simulink model "onelink_simscape"  (R2025a)
settings: Solver=ode15s  StartTime=0.0  StopTime=10  RelTol=1e-4
libraries: fl_lib x179, ee_lib x62, nesl_utility x15
(part 2 of 2)

== system onelink_simscape/inverter5 ==
  Electrical Reference1 : fl_lib/Electrical/Electrical Elements/Electrical Reference
  OP2 : ee_lib/Integrated Circuits/Band-Limited Op-Amp  A=1.8E6  Rin=4e6 Ohm  Rout=70 Ohm  Vmin=-24 V  Vmax=24 V  Vdotmax=2.8E6 V/s  f=8E6 Hz  V0=0 V
  m1 : fl_lib/Electrical/Electrical Elements/Resistor  R=1E3 Ohm  i_specify=off  i_priority=None  i=0 A  i_nominal_specify=off  i_nominal_value=1  i_nominal_unit=A  v_specify=off  v_priority=None  v=0 V  v_nominal_specify=off  v_nominal_value=1  v_nominal_unit=V
  m2 : fl_lib/Electrical/Electrical Elements/Resistor  R=1E3 Ohm  i_specify=off  i_priority=None  i=0 A  i_nominal_specify=off  i_nominal_value=1  i_nominal_unit=A  v_specify=off  v_priority=None  v=0 V  v_nominal_specify=off  v_nominal_value=1  v_nominal_unit=V
  in : PMIOPort  Side=Left
  out : PMIOPort  Port=2  Side=Right
  connections:
  m1/LConn1 -- in/RConn1
  out/RConn1 -- OP2/RConn1 -- m2/LConn1
  OP2/LConn2 -- m1/RConn1 -- m2/RConn1
  OP2/LConn1 -- Electrical Reference1/LConn1

== system onelink_simscape/inverter6 ==
  Electrical Reference1 : fl_lib/Electrical/Electrical Elements/Electrical Reference
  OP2 : ee_lib/Integrated Circuits/Band-Limited Op-Amp  A=1.8E6  Rin=4e6 Ohm  Rout=70 Ohm  Vmin=-24 V  Vmax=24 V  Vdotmax=2.8E6 V/s  f=8E6 Hz  V0=0 V
  m1 : fl_lib/Electrical/Electrical Elements/Resistor  R=1E3 Ohm  i_specify=off  i_priority=None  i=0 A  i_nominal_specify=off  i_nominal_value=1  i_nominal_unit=A  v_specify=off  v_priority=None  v=0 V  v_nominal_specify=off  v_nominal_value=1  v_nominal_unit=V
  m2 : fl_lib/Electrical/Electrical Elements/Resistor  R=1E3 Ohm  i_specify=off  i_priority=None  i=0 A  i_nominal_specify=off  i_nominal_value=1  i_nominal_unit=A  v_specify=off  v_priority=None  v=0 V  v_nominal_specify=off  v_nominal_value=1  v_nominal_unit=V
  in : PMIOPort  Side=Left
  out : PMIOPort  Port=2  Side=Right
  connections:
  m1/LConn1 -- in/RConn1
  out/RConn1 -- OP2/RConn1 -- m2/LConn1
  OP2/LConn2 -- m1/RConn1 -- m2/RConn1
  OP2/LConn1 -- Electrical Reference1/LConn1

== system onelink_simscape/inverter7 ==
  Electrical Reference1 : fl_lib/Electrical/Electrical Elements/Electrical Reference
  OP2 : ee_lib/Integrated Circuits/Band-Limited Op-Amp  A=1.8E6  Rin=4e6 Ohm  Rout=70 Ohm  Vmin=-24 V  Vmax=24 V  Vdotmax=2.8E6 V/s  f=8E6 Hz  V0=0 V
  m1 : fl_lib/Electrical/Electrical Elements/Resistor  R=1E3 Ohm  i_specify=off  i_priority=None  i=0 A  i_nominal_specify=off  i_nominal_value=1  i_nominal_unit=A  v_specify=off  v_priority=None  v=0 V  v_nominal_specify=off  v_nominal_value=1  v_nominal_unit=V
  m2 : fl_lib/Electrical/Electrical Elements/Resistor  R=1E3 Ohm  i_specify=off  i_priority=None  i=0 A  i_nominal_specify=off  i_nominal_value=1  i_nominal_unit=A  v_specify=off  v_priority=None  v=0 V  v_nominal_specify=off  v_nominal_value=1  v_nominal_unit=V
  in : PMIOPort  Side=Left
  out : PMIOPort  Port=2  Side=Right
  connections:
  m1/LConn1 -- in/RConn1
  out/RConn1 -- OP2/RConn1 -- m2/LConn1
  OP2/LConn2 -- m1/RConn1 -- m2/RConn1
  OP2/LConn1 -- Electrical Reference1/LConn1

== system onelink_simscape/inverter8 ==
  Electrical Reference1 : fl_lib/Electrical/Electrical Elements/Electrical Reference
  OP2 : ee_lib/Integrated Circuits/Band-Limited Op-Amp  A=1.8E6  Rin=4e6 Ohm  Rout=70 Ohm  Vmin=-24 V  Vmax=24 V  Vdotmax=2.8E6 V/s  f=8E6 Hz  V0=0 V
  m1 : fl_lib/Electrical/Electrical Elements/Resistor  R=1E3 Ohm  i_specify=off  i_priority=None  i=0 A  i_nominal_specify=off  i_nominal_value=1  i_nominal_unit=A  v_specify=off  v_priority=None  v=0 V  v_nominal_specify=off  v_nominal_value=1  v_nominal_unit=V
  m2 : fl_lib/Electrical/Electrical Elements/Resistor  R=1E3 Ohm  i_specify=off  i_priority=None  i=0 A  i_nominal_specify=off  i_nominal_value=1  i_nominal_unit=A  v_specify=off  v_priority=None  v=0 V  v_nominal_specify=off  v_nominal_value=1  v_nominal_unit=V
  in : PMIOPort  Side=Left
  out : PMIOPort  Port=2  Side=Right
  connections:
  m1/LConn1 -- in/RConn1
  out/RConn1 -- OP2/RConn1 -- m2/LConn1
  OP2/LConn2 -- m1/RConn1 -- m2/RConn1
  OP2/LConn1 -- Electrical Reference1/LConn1

== system onelink_simscape/inverter9 ==
  Electrical Reference1 : fl_lib/Electrical/Electrical Elements/Electrical Reference
  OP2 : ee_lib/Integrated Circuits/Band-Limited Op-Amp  A=1.8E6  Rin=4e6 Ohm  Rout=70 Ohm  Vmin=-24 V  Vmax=24 V  Vdotmax=2.8E6 V/s  f=8E6 Hz  V0=0 V
  m1 : fl_lib/Electrical/Electrical Elements/Resistor  R=1E3 Ohm  i_specify=off  i_priority=None  i=0 A  i_nominal_specify=off  i_nominal_value=1  i_nominal_unit=A  v_specify=off  v_priority=None  v=0 V  v_nominal_specify=off  v_nominal_value=1  v_nominal_unit=V
  m2 : fl_lib/Electrical/Electrical Elements/Resistor  R=1E3 Ohm  i_specify=off  i_priority=None  i=0 A  i_nominal_specify=off  i_nominal_value=1  i_nominal_unit=A  v_specify=off  v_priority=None  v=0 V  v_nominal_specify=off  v_nominal_value=1  v_nominal_unit=V
  in : PMIOPort  Side=Left
  out : PMIOPort  Port=2  Side=Right
  connections:
  m1/LConn1 -- in/RConn1
  out/RConn1 -- OP2/RConn1 -- m2/LConn1
  OP2/LConn2 -- m1/RConn1 -- m2/RConn1
  OP2/LConn1 -- Electrical Reference1/LConn1

== system onelink_simscape/mulitplier1 ==
  note: Multiplication circuit. The output voltage is
      | Vx * Vy / K where Multiplier block
      | parameter K is the scaling factor.
  ERef M1Y1 : fl_lib/Electrical/Electrical Elements/Electrical Reference
  ERef M1Y2 : fl_lib/Electrical/Electrical Elements/Electrical Reference
  ERef M1Z2 : fl_lib/Electrical/Electrical Elements/Electrical Reference
  Multiplier 1 : ee_lib/Integrated Circuits/Multiplier  K=1 V  A=3e+3  Rin=1e+7 Ohm  Vdiff=24 V  Rout=0.1 Ohm  Vmin=-11 V  Vmax=11 V  Vdotmax=20 V/us  f=1 MHz  V0=0 V
      settings: AttributesFormatString=Scaling Factor = %<K>  InternalSimscapePortConfiguration="{\"Bottom\":[],\"Left\":[{\"id\":\"X1\",\"label\":\"X1\",\"type\":\"foundation.electrical.electrical\"},{\"id\":\"X2\",\"label\":\"X2\",\"type\":\"foundation.electrical.electrical\"},{\"id\":\"Y1\",\"label\":\"Y1\",\"type\":\"foundation.electrical.electrical\"},{\"id\":\"Y2\",\"label\":\"Y2\",\"type\":\"foundation.electrical.electrical\"},{\"id\":\"Z1\",\"label\":\"Z1\",\"type\":\"foundation.electrical.electrical\"},{\"id\":\"Z2\",\"label\":\"Z2\",\"type\":\"foundation.electrical.electrical\"}],\"Right\":[{\"id\":\"out\",\"label\":\"\",\"type\":\"foundation.electrical.electrical\"}],\"Top\":[]}"
  in1 : PMIOPort  Side=Left
  in2 : PMIOPort  Port=2  Side=Left
  out : PMIOPort  Port=3  Side=Right
  connections:
  Multiplier 1/RConn1 -- out/RConn1 -- Multiplier 1/LConn5
  ERef M1Z2/LConn1 -- Multiplier 1/LConn6
  ERef M1Y2/LConn1 -- Multiplier 1/LConn4
  Multiplier 1/LConn3 -- in2/RConn1
  Multiplier 1/LConn2 -- ERef M1Y1/LConn1
  Multiplier 1/LConn1 -- in1/RConn1

== system onelink_simscape/mulitplier10 ==
  note: Multiplication circuit. The output voltage is
      | Vx * Vy / K where Multiplier block
      | parameter K is the scaling factor.
  ERef M1Y1 : fl_lib/Electrical/Electrical Elements/Electrical Reference
  ERef M1Y2 : fl_lib/Electrical/Electrical Elements/Electrical Reference
  ERef M1Z2 : fl_lib/Electrical/Electrical Elements/Electrical Reference
  Multiplier 1 : ee_lib/Integrated Circuits/Multiplier  K=1 V  A=3e+3  Rin=1e+7 Ohm  Vdiff=10 V  Rout=0.1 Ohm  Vmin=-11 V  Vmax=11 V  Vdotmax=20 V/us  f=1 MHz  V0=0 V
      settings: AttributesFormatString=Scaling Factor = %<K>  InternalSimscapePortConfiguration="{\"Bottom\":[],\"Left\":[{\"id\":\"X1\",\"label\":\"X1\",\"type\":\"foundation.electrical.electrical\"},{\"id\":\"X2\",\"label\":\"X2\",\"type\":\"foundation.electrical.electrical\"},{\"id\":\"Y1\",\"label\":\"Y1\",\"type\":\"foundation.electrical.electrical\"},{\"id\":\"Y2\",\"label\":\"Y2\",\"type\":\"foundation.electrical.electrical\"},{\"id\":\"Z1\",\"label\":\"Z1\",\"type\":\"foundation.electrical.electrical\"},{\"id\":\"Z2\",\"label\":\"Z2\",\"type\":\"foundation.electrical.electrical\"}],\"Right\":[{\"id\":\"out\",\"label\":\"\",\"type\":\"foundation.electrical.electrical\"}],\"Top\":[]}"
  in1 : PMIOPort  Side=Left
  in2 : PMIOPort  Port=2  Side=Left
  out : PMIOPort  Port=3  Side=Right
  connections:
  Multiplier 1/RConn1 -- out/RConn1 -- Multiplier 1/LConn5
  ERef M1Z2/LConn1 -- Multiplier 1/LConn6
  ERef M1Y2/LConn1 -- Multiplier 1/LConn4
  Multiplier 1/LConn3 -- in2/RConn1
  Multiplier 1/LConn2 -- ERef M1Y1/LConn1
  Multiplier 1/LConn1 -- in1/RConn1

== system onelink_simscape/mulitplier11 ==
  note: Multiplication circuit. The output voltage is
      | Vx * Vy / K where Multiplier block
      | parameter K is the scaling factor.
  ERef M1Y1 : fl_lib/Electrical/Electrical Elements/Electrical Reference
  ERef M1Y2 : fl_lib/Electrical/Electrical Elements/Electrical Reference
  ERef M1Z2 : fl_lib/Electrical/Electrical Elements/Electrical Reference
  Multiplier 1 : ee_lib/Integrated Circuits/Multiplier  K=1 V  A=3e+3  Rin=1e+7 Ohm  Vdiff=10 V  Rout=0.1 Ohm  Vmin=-11 V  Vmax=11 V  Vdotmax=20 V/us  f=1 MHz  V0=0 V
      settings: AttributesFormatString=Scaling Factor = %<K>  InternalSimscapePortConfiguration="{\"Bottom\":[],\"Left\":[{\"id\":\"X1\",\"label\":\"X1\",\"type\":\"foundation.electrical.electrical\"},{\"id\":\"X2\",\"label\":\"X2\",\"type\":\"foundation.electrical.electrical\"},{\"id\":\"Y1\",\"label\":\"Y1\",\"type\":\"foundation.electrical.electrical\"},{\"id\":\"Y2\",\"label\":\"Y2\",\"type\":\"foundation.electrical.electrical\"},{\"id\":\"Z1\",\"label\":\"Z1\",\"type\":\"foundation.electrical.electrical\"},{\"id\":\"Z2\",\"label\":\"Z2\",\"type\":\"foundation.electrical.electrical\"}],\"Right\":[{\"id\":\"out\",\"label\":\"\",\"type\":\"foundation.electrical.electrical\"}],\"Top\":[]}"
  in1 : PMIOPort  Side=Left
  in2 : PMIOPort  Port=2  Side=Left
  out : PMIOPort  Port=3  Side=Right
  connections:
  Multiplier 1/RConn1 -- out/RConn1 -- Multiplier 1/LConn5
  ERef M1Z2/LConn1 -- Multiplier 1/LConn6
  ERef M1Y2/LConn1 -- Multiplier 1/LConn4
  Multiplier 1/LConn3 -- in2/RConn1
  Multiplier 1/LConn2 -- ERef M1Y1/LConn1
  Multiplier 1/LConn1 -- in1/RConn1

== system onelink_simscape/mulitplier2 ==
  note: Multiplication circuit. The output voltage is
      | Vx * Vy / K where Multiplier block
      | parameter K is the scaling factor.
  ERef M1Y1 : fl_lib/Electrical/Electrical Elements/Electrical Reference
  ERef M1Y2 : fl_lib/Electrical/Electrical Elements/Electrical Reference
  ERef M1Z2 : fl_lib/Electrical/Electrical Elements/Electrical Reference
  Multiplier 1 : ee_lib/Integrated Circuits/Multiplier  K=1 V  A=3e+3  Rin=1e+7 Ohm  Vdiff=24 V  Rout=0.1 Ohm  Vmin=-11 V  Vmax=11 V  Vdotmax=20 V/us  f=1 MHz  V0=0 V
      settings: AttributesFormatString=Scaling Factor = %<K>  InternalSimscapePortConfiguration="{\"Bottom\":[],\"Left\":[{\"id\":\"X1\",\"label\":\"X1\",\"type\":\"foundation.electrical.electrical\"},{\"id\":\"X2\",\"label\":\"X2\",\"type\":\"foundation.electrical.electrical\"},{\"id\":\"Y1\",\"label\":\"Y1\",\"type\":\"foundation.electrical.electrical\"},{\"id\":\"Y2\",\"label\":\"Y2\",\"type\":\"foundation.electrical.electrical\"},{\"id\":\"Z1\",\"label\":\"Z1\",\"type\":\"foundation.electrical.electrical\"},{\"id\":\"Z2\",\"label\":\"Z2\",\"type\":\"foundation.electrical.electrical\"}],\"Right\":[{\"id\":\"out\",\"label\":\"\",\"type\":\"foundation.electrical.electrical\"}],\"Top\":[]}"
  in1 : PMIOPort  Side=Left
  in2 : PMIOPort  Port=2  Side=Left
  out : PMIOPort  Port=3  Side=Right
  connections:
  Multiplier 1/RConn1 -- out/RConn1 -- Multiplier 1/LConn5
  ERef M1Z2/LConn1 -- Multiplier 1/LConn6
  ERef M1Y2/LConn1 -- Multiplier 1/LConn4
  Multiplier 1/LConn3 -- in2/RConn1
  Multiplier 1/LConn2 -- ERef M1Y1/LConn1
  Multiplier 1/LConn1 -- in1/RConn1

== system onelink_simscape/mulitplier3 ==
  note: Multiplication circuit. The output voltage is
      | Vx * Vy / K where Multiplier block
      | parameter K is the scaling factor.
  ERef M1Y1 : fl_lib/Electrical/Electrical Elements/Electrical Reference
  ERef M1Y2 : fl_lib/Electrical/Electrical Elements/Electrical Reference
  ERef M1Z2 : fl_lib/Electrical/Electrical Elements/Electrical Reference
  Multiplier 1 : ee_lib/Integrated Circuits/Multiplier  K=1 V  A=3e+3  Rin=1e+7 Ohm  Vdiff=24 V  Rout=0.1 Ohm  Vmin=-18 V  Vmax=18 V  Vdotmax=20 V/us  f=1 MHz  V0=0 V
      settings: AttributesFormatString=Scaling Factor = %<K>  InternalSimscapePortConfiguration="{\"Bottom\":[],\"Left\":[{\"id\":\"X1\",\"label\":\"X1\",\"type\":\"foundation.electrical.electrical\"},{\"id\":\"X2\",\"label\":\"X2\",\"type\":\"foundation.electrical.electrical\"},{\"id\":\"Y1\",\"label\":\"Y1\",\"type\":\"foundation.electrical.electrical\"},{\"id\":\"Y2\",\"label\":\"Y2\",\"type\":\"foundation.electrical.electrical\"},{\"id\":\"Z1\",\"label\":\"Z1\",\"type\":\"foundation.electrical.electrical\"},{\"id\":\"Z2\",\"label\":\"Z2\",\"type\":\"foundation.electrical.electrical\"}],\"Right\":[{\"id\":\"out\",\"label\":\"\",\"type\":\"foundation.electrical.electrical\"}],\"Top\":[]}"
  in1 : PMIOPort  Side=Left
  in2 : PMIOPort  Port=2  Side=Left
  out : PMIOPort  Port=3  Side=Right
  connections:
  Multiplier 1/RConn1 -- out/RConn1 -- Multiplier 1/LConn5
  ERef M1Z2/LConn1 -- Multiplier 1/LConn6
  ERef M1Y2/LConn1 -- Multiplier 1/LConn4
  Multiplier 1/LConn3 -- in2/RConn1
  Multiplier 1/LConn2 -- ERef M1Y1/LConn1
  Multiplier 1/LConn1 -- in1/RConn1

== system onelink_simscape/mulitplier4 ==
  note: Multiplication circuit. The output voltage is
      | Vx * Vy / K where Multiplier block
      | parameter K is the scaling factor.
  ERef M1Y1 : fl_lib/Electrical/Electrical Elements/Electrical Reference
  ERef M1Y2 : fl_lib/Electrical/Electrical Elements/Electrical Reference
  ERef M1Z2 : fl_lib/Electrical/Electrical Elements/Electrical Reference
  Multiplier 1 : ee_lib/Integrated Circuits/Multiplier  K=1 V  A=3e+3  Rin=1e+7 Ohm  Vdiff=24 V  Rout=0.1 Ohm  Vmin=-11 V  Vmax=11 V  Vdotmax=20 V/us  f=1 MHz  V0=0 V
      settings: AttributesFormatString=Scaling Factor = %<K>  InternalSimscapePortConfiguration="{\"Bottom\":[],\"Left\":[{\"id\":\"X1\",\"label\":\"X1\",\"type\":\"foundation.electrical.electrical\"},{\"id\":\"X2\",\"label\":\"X2\",\"type\":\"foundation.electrical.electrical\"},{\"id\":\"Y1\",\"label\":\"Y1\",\"type\":\"foundation.electrical.electrical\"},{\"id\":\"Y2\",\"label\":\"Y2\",\"type\":\"foundation.electrical.electrical\"},{\"id\":\"Z1\",\"label\":\"Z1\",\"type\":\"foundation.electrical.electrical\"},{\"id\":\"Z2\",\"label\":\"Z2\",\"type\":\"foundation.electrical.electrical\"}],\"Right\":[{\"id\":\"out\",\"label\":\"\",\"type\":\"foundation.electrical.electrical\"}],\"Top\":[]}"
  in1 : PMIOPort  Side=Left
  in2 : PMIOPort  Port=2  Side=Left
  out : PMIOPort  Port=3  Side=Right
  connections:
  Multiplier 1/RConn1 -- out/RConn1 -- Multiplier 1/LConn5
  ERef M1Z2/LConn1 -- Multiplier 1/LConn6
  ERef M1Y2/LConn1 -- Multiplier 1/LConn4
  Multiplier 1/LConn3 -- in2/RConn1
  Multiplier 1/LConn2 -- ERef M1Y1/LConn1
  Multiplier 1/LConn1 -- in1/RConn1

== system onelink_simscape/mulitplier5 ==
  note: Multiplication circuit. The output voltage is
      | Vx * Vy / K where Multiplier block
      | parameter K is the scaling factor.
  ERef M1Y1 : fl_lib/Electrical/Electrical Elements/Electrical Reference
  ERef M1Y2 : fl_lib/Electrical/Electrical Elements/Electrical Reference
  ERef M1Z2 : fl_lib/Electrical/Electrical Elements/Electrical Reference
  Multiplier 1 : ee_lib/Integrated Circuits/Multiplier  K=1 V  A=3e+3  Rin=1e+7 Ohm  Vdiff=24 V  Rout=0.1 Ohm  Vmin=-11 V  Vmax=11 V  Vdotmax=20 V/us  f=1 MHz  V0=0 V
      settings: AttributesFormatString=Scaling Factor = %<K>  InternalSimscapePortConfiguration="{\"Bottom\":[],\"Left\":[{\"id\":\"X1\",\"label\":\"X1\",\"type\":\"foundation.electrical.electrical\"},{\"id\":\"X2\",\"label\":\"X2\",\"type\":\"foundation.electrical.electrical\"},{\"id\":\"Y1\",\"label\":\"Y1\",\"type\":\"foundation.electrical.electrical\"},{\"id\":\"Y2\",\"label\":\"Y2\",\"type\":\"foundation.electrical.electrical\"},{\"id\":\"Z1\",\"label\":\"Z1\",\"type\":\"foundation.electrical.electrical\"},{\"id\":\"Z2\",\"label\":\"Z2\",\"type\":\"foundation.electrical.electrical\"}],\"Right\":[{\"id\":\"out\",\"label\":\"\",\"type\":\"foundation.electrical.electrical\"}],\"Top\":[]}"
  in1 : PMIOPort  Side=Left
  in2 : PMIOPort  Port=2  Side=Left
  out : PMIOPort  Port=3  Side=Right
  connections:
  Multiplier 1/RConn1 -- out/RConn1 -- Multiplier 1/LConn5
  ERef M1Z2/LConn1 -- Multiplier 1/LConn6
  ERef M1Y2/LConn1 -- Multiplier 1/LConn4
  Multiplier 1/LConn3 -- in2/RConn1
  Multiplier 1/LConn2 -- ERef M1Y1/LConn1
  Multiplier 1/LConn1 -- in1/RConn1

== system onelink_simscape/mulitplier6 ==
  note: Multiplication circuit. The output voltage is
      | Vx * Vy / K where Multiplier block
      | parameter K is the scaling factor.
  ERef M1Y1 : fl_lib/Electrical/Electrical Elements/Electrical Reference
  ERef M1Y2 : fl_lib/Electrical/Electrical Elements/Electrical Reference
  ERef M1Z2 : fl_lib/Electrical/Electrical Elements/Electrical Reference
  Multiplier 1 : ee_lib/Integrated Circuits/Multiplier  K=1 V  A=3e+3  Rin=1e+7 Ohm  Vdiff=24 V  Rout=0.1 Ohm  Vmin=-11 V  Vmax=11 V  Vdotmax=20 V/us  f=1 MHz  V0=0 V
      settings: AttributesFormatString=Scaling Factor = %<K>  InternalSimscapePortConfiguration="{\"Bottom\":[],\"Left\":[{\"id\":\"X1\",\"label\":\"X1\",\"type\":\"foundation.electrical.electrical\"},{\"id\":\"X2\",\"label\":\"X2\",\"type\":\"foundation.electrical.electrical\"},{\"id\":\"Y1\",\"label\":\"Y1\",\"type\":\"foundation.electrical.electrical\"},{\"id\":\"Y2\",\"label\":\"Y2\",\"type\":\"foundation.electrical.electrical\"},{\"id\":\"Z1\",\"label\":\"Z1\",\"type\":\"foundation.electrical.electrical\"},{\"id\":\"Z2\",\"label\":\"Z2\",\"type\":\"foundation.electrical.electrical\"}],\"Right\":[{\"id\":\"out\",\"label\":\"\",\"type\":\"foundation.electrical.electrical\"}],\"Top\":[]}"
  in1 : PMIOPort  Side=Left
  in2 : PMIOPort  Port=2  Side=Left
  out : PMIOPort  Port=3  Side=Right
  connections:
  Multiplier 1/RConn1 -- out/RConn1 -- Multiplier 1/LConn5
  ERef M1Z2/LConn1 -- Multiplier 1/LConn6
  ERef M1Y2/LConn1 -- Multiplier 1/LConn4
  Multiplier 1/LConn3 -- in2/RConn1
  Multiplier 1/LConn2 -- ERef M1Y1/LConn1
  Multiplier 1/LConn1 -- in1/RConn1

== system onelink_simscape/mulitplier7 ==
  note: Multiplication circuit. The output voltage is
      | Vx * Vy / K where Multiplier block
      | parameter K is the scaling factor.
  ERef M1Y1 : fl_lib/Electrical/Electrical Elements/Electrical Reference
  ERef M1Y2 : fl_lib/Electrical/Electrical Elements/Electrical Reference
  ERef M1Z2 : fl_lib/Electrical/Electrical Elements/Electrical Reference
  Multiplier 1 : ee_lib/Integrated Circuits/Multiplier  K=1 V  A=3e+3  Rin=1e+7 Ohm  Vdiff=24 V  Rout=0.1 Ohm  Vmin=-11 V  Vmax=11 V  Vdotmax=20 V/us  f=1 MHz  V0=0 V
      settings: AttributesFormatString=Scaling Factor = %<K>  InternalSimscapePortConfiguration="{\"Bottom\":[],\"Left\":[{\"id\":\"X1\",\"label\":\"X1\",\"type\":\"foundation.electrical.electrical\"},{\"id\":\"X2\",\"label\":\"X2\",\"type\":\"foundation.electrical.electrical\"},{\"id\":\"Y1\",\"label\":\"Y1\",\"type\":\"foundation.electrical.electrical\"},{\"id\":\"Y2\",\"label\":\"Y2\",\"type\":\"foundation.electrical.electrical\"},{\"id\":\"Z1\",\"label\":\"Z1\",\"type\":\"foundation.electrical.electrical\"},{\"id\":\"Z2\",\"label\":\"Z2\",\"type\":\"foundation.electrical.electrical\"}],\"Right\":[{\"id\":\"out\",\"label\":\"\",\"type\":\"foundation.electrical.electrical\"}],\"Top\":[]}"
  in1 : PMIOPort  Side=Left
  in2 : PMIOPort  Port=2  Side=Left
  out : PMIOPort  Port=3  Side=Right
  connections:
  Multiplier 1/RConn1 -- out/RConn1 -- Multiplier 1/LConn5
  ERef M1Z2/LConn1 -- Multiplier 1/LConn6
  ERef M1Y2/LConn1 -- Multiplier 1/LConn4
  Multiplier 1/LConn3 -- in2/RConn1
  Multiplier 1/LConn2 -- ERef M1Y1/LConn1
  Multiplier 1/LConn1 -- in1/RConn1

== system onelink_simscape/mulitplier8 ==
  note: Multiplication circuit. The output voltage is
      | Vx * Vy / K where Multiplier block
      | parameter K is the scaling factor.
  ERef M1Y1 : fl_lib/Electrical/Electrical Elements/Electrical Reference
  ERef M1Y2 : fl_lib/Electrical/Electrical Elements/Electrical Reference
  ERef M1Z2 : fl_lib/Electrical/Electrical Elements/Electrical Reference
  Multiplier 1 : ee_lib/Integrated Circuits/Multiplier  K=1 V  A=3e+3  Rin=1e+7 Ohm  Vdiff=24 V  Rout=0.1 Ohm  Vmin=-11 V  Vmax=11 V  Vdotmax=20 V/us  f=1 MHz  V0=0 V
      settings: AttributesFormatString=Scaling Factor = %<K>  InternalSimscapePortConfiguration="{\"Bottom\":[],\"Left\":[{\"id\":\"X1\",\"label\":\"X1\",\"type\":\"foundation.electrical.electrical\"},{\"id\":\"X2\",\"label\":\"X2\",\"type\":\"foundation.electrical.electrical\"},{\"id\":\"Y1\",\"label\":\"Y1\",\"type\":\"foundation.electrical.electrical\"},{\"id\":\"Y2\",\"label\":\"Y2\",\"type\":\"foundation.electrical.electrical\"},{\"id\":\"Z1\",\"label\":\"Z1\",\"type\":\"foundation.electrical.electrical\"},{\"id\":\"Z2\",\"label\":\"Z2\",\"type\":\"foundation.electrical.electrical\"}],\"Right\":[{\"id\":\"out\",\"label\":\"\",\"type\":\"foundation.electrical.electrical\"}],\"Top\":[]}"
  in1 : PMIOPort  Side=Left
  in2 : PMIOPort  Port=2  Side=Left
  out : PMIOPort  Port=3  Side=Right
  connections:
  Multiplier 1/RConn1 -- out/RConn1 -- Multiplier 1/LConn5
  ERef M1Z2/LConn1 -- Multiplier 1/LConn6
  ERef M1Y2/LConn1 -- Multiplier 1/LConn4
  Multiplier 1/LConn3 -- in2/RConn1
  Multiplier 1/LConn2 -- ERef M1Y1/LConn1
  Multiplier 1/LConn1 -- in1/RConn1

== system onelink_simscape/mulitplier9 ==
  note: Multiplication circuit. The output voltage is
      | Vx * Vy / K where Multiplier block
      | parameter K is the scaling factor.
  ERef M1Y1 : fl_lib/Electrical/Electrical Elements/Electrical Reference
  ERef M1Y2 : fl_lib/Electrical/Electrical Elements/Electrical Reference
  ERef M1Z2 : fl_lib/Electrical/Electrical Elements/Electrical Reference
  Multiplier 1 : ee_lib/Integrated Circuits/Multiplier  K=1 V  A=3e+3  Rin=1e+7 Ohm  Vdiff=24 V  Rout=0.1 Ohm  Vmin=-11 V  Vmax=11 V  Vdotmax=20 V/us  f=1 MHz  V0=0 V
      settings: AttributesFormatString=Scaling Factor = %<K>  InternalSimscapePortConfiguration="{\"Bottom\":[],\"Left\":[{\"id\":\"X1\",\"label\":\"X1\",\"type\":\"foundation.electrical.electrical\"},{\"id\":\"X2\",\"label\":\"X2\",\"type\":\"foundation.electrical.electrical\"},{\"id\":\"Y1\",\"label\":\"Y1\",\"type\":\"foundation.electrical.electrical\"},{\"id\":\"Y2\",\"label\":\"Y2\",\"type\":\"foundation.electrical.electrical\"},{\"id\":\"Z1\",\"label\":\"Z1\",\"type\":\"foundation.electrical.electrical\"},{\"id\":\"Z2\",\"label\":\"Z2\",\"type\":\"foundation.electrical.electrical\"}],\"Right\":[{\"id\":\"out\",\"label\":\"\",\"type\":\"foundation.electrical.electrical\"}],\"Top\":[]}"
  in1 : PMIOPort  Side=Left
  in2 : PMIOPort  Port=2  Side=Left
  out : PMIOPort  Port=3  Side=Right
  connections:
  Multiplier 1/RConn1 -- out/RConn1 -- Multiplier 1/LConn5
  ERef M1Z2/LConn1 -- Multiplier 1/LConn6
  ERef M1Y2/LConn1 -- Multiplier 1/LConn4
  Multiplier 1/LConn3 -- in2/RConn1
  Multiplier 1/LConn2 -- ERef M1Y1/LConn1
  Multiplier 1/LConn1 -- in1/RConn1

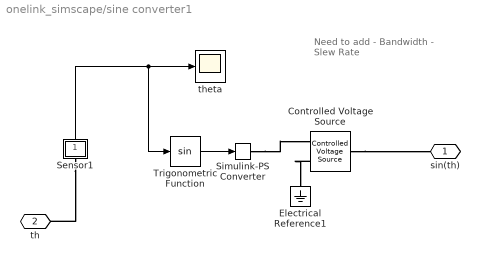
== system onelink_simscape/sine converter1 ==
  note: Need to add
      | - Bandwidth
      | - Slew Rate
  Controlled Voltage Source : fl_lib/Electrical/Electrical Sources/Controlled Voltage Source
  Electrical Reference1 : fl_lib/Electrical/Electrical Elements/Electrical Reference
  Sensor1 : Subsystem
      mask Display: disp('S')
  Simulink-PS Converter : nesl_utility/Simulink-PS Converter  PhysicalDomain=network_engine_domain  SubClassName=ps_input  LeftPortType=input  RightPortType=output  PseudoPeriodic=off  Frequencies=[]  NoiseDistribution=none  NoiseParameters=[]  Unit=1  AffineConversion=off  FilteringAndDerivatives=provide  SimscapeFilterOrder=1  InputFilterTimeConstant=0.001  UdotUserProvided=0
  Trigonometric Function : Trigonometry
  theta : Scope
      settings: ActiveDisplayYMinimum=-0.06401  ActiveDisplayYMaximum=0.47536  DataLoggingVariableName=ScopeData2
  sin(th) : PMIOPort  Side=Right
  th : PMIOPort  Port=2  Side=Left
  wires:
  Trigonometric Function/1 -> Simulink-PS Converter/1
  Sensor1/1(Out1) -> theta/1, Trigonometric Function/1
  connections:
  Controlled Voltage Source/LConn1 -- sin(th)/RConn1
  Sensor1/LConn1 -- th/RConn1
  Simulink-PS Converter/RConn1 -- Controlled Voltage Source/RConn1
  Controlled Voltage Source/RConn2 -- Electrical Reference1/LConn1

== system onelink_simscape/square4 ==
  note: Multiplication circuit. The output voltage is
      | Vx * Vy / K where Multiplier block
      | parameter K is the scaling factor.
  ERef M1Y1 : fl_lib/Electrical/Electrical Elements/Electrical Reference
  ERef M1Y2 : fl_lib/Electrical/Electrical Elements/Electrical Reference
  ERef M1Z2 : fl_lib/Electrical/Electrical Elements/Electrical Reference
  Multiplier 1 : ee_lib/Integrated Circuits/Multiplier  K=1 V  A=3e+3  Rin=1e+7 Ohm  Vdiff=10 V  Rout=0.1 Ohm  Vmin=-18 V  Vmax=18 V  Vdotmax=20 V/us  f=1 MHz  V0=0 V
      settings: AttributesFormatString=Scaling Factor = %<K>  InternalSimscapePortConfiguration="{\"Bottom\":[],\"Left\":[{\"id\":\"X1\",\"label\":\"X1\",\"type\":\"foundation.electrical.electrical\"},{\"id\":\"X2\",\"label\":\"X2\",\"type\":\"foundation.electrical.electrical\"},{\"id\":\"Y1\",\"label\":\"Y1\",\"type\":\"foundation.electrical.electrical\"},{\"id\":\"Y2\",\"label\":\"Y2\",\"type\":\"foundation.electrical.electrical\"},{\"id\":\"Z1\",\"label\":\"Z1\",\"type\":\"foundation.electrical.electrical\"},{\"id\":\"Z2\",\"label\":\"Z2\",\"type\":\"foundation.electrical.electrical\"}],\"Right\":[{\"id\":\"out\",\"label\":\"\",\"type\":\"foundation.electrical.electrical\"}],\"Top\":[]}"
  in1 : PMIOPort  Side=Left
  in2 : PMIOPort  Port=2  Side=Left
  out : PMIOPort  Port=3  Side=Right
  connections:
  Multiplier 1/LConn5 -- Multiplier 1/RConn1 -- out/RConn1
  ERef M1Z2/LConn1 -- Multiplier 1/LConn6
  ERef M1Y2/LConn1 -- Multiplier 1/LConn4
  Multiplier 1/LConn3 -- in2/RConn1
  Multiplier 1/LConn2 -- ERef M1Y1/LConn1
  Multiplier 1/LConn1 -- in1/RConn1

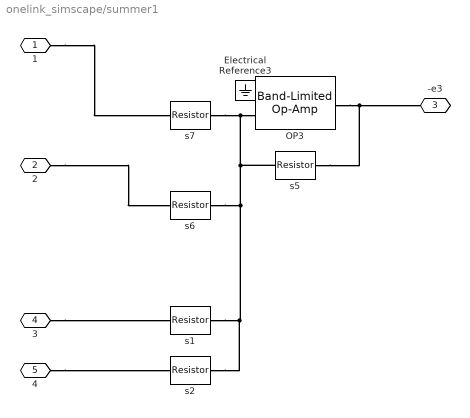
== system onelink_simscape/summer1 ==
  Electrical Reference3 : fl_lib/Electrical/Electrical Elements/Electrical Reference
  OP3 : ee_lib/Integrated Circuits/Band-Limited Op-Amp  A=1.8E6  Rin=4e6 Ohm  Rout=70 Ohm  Vmin=-24 V  Vmax=24 V  Vdotmax=2.8E6 V/s  f=8E6 Hz  V0=0 V
  s{1..2,5..7} (5 alike) : fl_lib/Electrical/Electrical Elements/Resistor  R=10E3 Ohm  i_specify=off  i_priority=None  i=0 A  i_nominal_specify=off  i_nominal_value=1  i_nominal_unit=A  v_specify=off  v_priority=None  v=0 V  v_nominal_specify=off  v_nominal_value=1  v_nominal_unit=V
  1 : PMIOPort  Side=Left
  2 : PMIOPort  Port=2  Side=Left
  -e3 : PMIOPort  Port=3  Side=Right
  3 : PMIOPort  Port=4  Side=Left
  4 : PMIOPort  Port=5  Side=Left
  connections:
  3/RConn1 -- s1/LConn1
  s2/RConn1 -- s1/RConn1 -- s6/RConn1 -- s5/LConn1 -- s7/RConn1 -- OP3/LConn2
  OP3/RConn1 -- -e3/RConn1 -- s5/RConn1
  Electrical Reference3/LConn1 -- OP3/LConn1
  2/RConn1 -- s6/LConn1
  1/RConn1 -- s7/LConn1
  4/RConn1 -- s2/LConn1

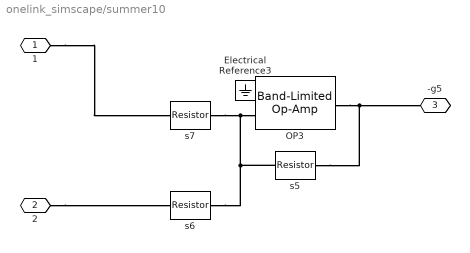
== system onelink_simscape/summer10 ==
  Electrical Reference3 : fl_lib/Electrical/Electrical Elements/Electrical Reference
  OP3 : ee_lib/Integrated Circuits/Band-Limited Op-Amp  A=1.8E6  Rin=4e6 Ohm  Rout=70 Ohm  Vmin=-24 V  Vmax=24 V  Vdotmax=2.8E6 V/s  f=8E6 Hz  V0=0 V
  s5 : fl_lib/Electrical/Electrical Elements/Resistor  R=10E3 Ohm  i_specify=off  i_priority=None  i=0 A  i_nominal_specify=off  i_nominal_value=1  i_nominal_unit=A  v_specify=off  v_priority=None  v=0 V  v_nominal_specify=off  v_nominal_value=1  v_nominal_unit=V
  s6 : fl_lib/Electrical/Electrical Elements/Resistor  R=10E3 Ohm  i_specify=off  i_priority=None  i=0 A  i_nominal_specify=off  i_nominal_value=1  i_nominal_unit=A  v_specify=off  v_priority=None  v=0 V  v_nominal_specify=off  v_nominal_value=1  v_nominal_unit=V
  s7 : fl_lib/Electrical/Electrical Elements/Resistor  R=10E3 Ohm  i_specify=off  i_priority=None  i=0 A  i_nominal_specify=off  i_nominal_value=1  i_nominal_unit=A  v_specify=off  v_priority=None  v=0 V  v_nominal_specify=off  v_nominal_value=1  v_nominal_unit=V
  1 : PMIOPort  Side=Left
  2 : PMIOPort  Port=2  Side=Left
  -g5 : PMIOPort  Port=3  Side=Right
  connections:
  s6/RConn1 -- s5/LConn1 -- s7/RConn1 -- OP3/LConn2
  OP3/RConn1 -- -g5/RConn1 -- s5/RConn1
  Electrical Reference3/LConn1 -- OP3/LConn1
  2/RConn1 -- s6/LConn1
  1/RConn1 -- s7/LConn1

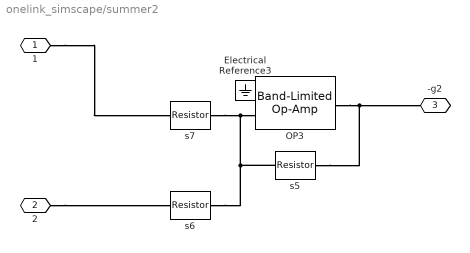
== system onelink_simscape/summer2 ==
  Electrical Reference3 : fl_lib/Electrical/Electrical Elements/Electrical Reference
  OP3 : ee_lib/Integrated Circuits/Band-Limited Op-Amp  A=1.8E6  Rin=4e6 Ohm  Rout=70 Ohm  Vmin=-24 V  Vmax=24 V  Vdotmax=2.8E6 V/s  f=8E6 Hz  V0=0 V
  s5 : fl_lib/Electrical/Electrical Elements/Resistor  R=10E3 Ohm  i_specify=off  i_priority=None  i=0 A  i_nominal_specify=off  i_nominal_value=1  i_nominal_unit=A  v_specify=off  v_priority=None  v=0 V  v_nominal_specify=off  v_nominal_value=1  v_nominal_unit=V
  s6 : fl_lib/Electrical/Electrical Elements/Resistor  R=10E3 Ohm  i_specify=off  i_priority=None  i=0 A  i_nominal_specify=off  i_nominal_value=1  i_nominal_unit=A  v_specify=off  v_priority=None  v=0 V  v_nominal_specify=off  v_nominal_value=1  v_nominal_unit=V
  s7 : fl_lib/Electrical/Electrical Elements/Resistor  R=10E3 Ohm  i_specify=off  i_priority=None  i=0 A  i_nominal_specify=off  i_nominal_value=1  i_nominal_unit=A  v_specify=off  v_priority=None  v=0 V  v_nominal_specify=off  v_nominal_value=1  v_nominal_unit=V
  1 : PMIOPort  Side=Left
  2 : PMIOPort  Port=2  Side=Left
  -g2 : PMIOPort  Port=3  Side=Right
  connections:
  s6/RConn1 -- s5/LConn1 -- s7/RConn1 -- OP3/LConn2
  OP3/RConn1 -- -g2/RConn1 -- s5/RConn1
  Electrical Reference3/LConn1 -- OP3/LConn1
  2/RConn1 -- s6/LConn1
  1/RConn1 -- s7/LConn1

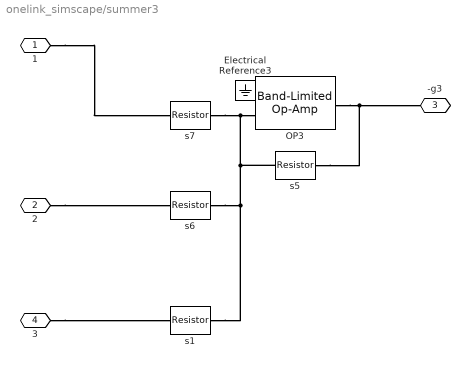
== system onelink_simscape/summer3 ==
  Electrical Reference3 : fl_lib/Electrical/Electrical Elements/Electrical Reference
  OP3 : ee_lib/Integrated Circuits/Band-Limited Op-Amp  A=1.8E6  Rin=4e6 Ohm  Rout=70 Ohm  Vmin=-24 V  Vmax=24 V  Vdotmax=2.8E6 V/s  f=8E6 Hz  V0=0 V
  s{1,5..7} (4 alike) : fl_lib/Electrical/Electrical Elements/Resistor  R=10E3 Ohm  i_specify=off  i_priority=None  i=0 A  i_nominal_specify=off  i_nominal_value=1  i_nominal_unit=A  v_specify=off  v_priority=None  v=0 V  v_nominal_specify=off  v_nominal_value=1  v_nominal_unit=V
  1 : PMIOPort  Side=Left
  2 : PMIOPort  Port=2  Side=Left
  -g3 : PMIOPort  Port=3  Side=Right
  3 : PMIOPort  Port=4  Side=Left
  connections:
  3/RConn1 -- s1/LConn1
  s1/RConn1 -- s6/RConn1 -- s5/LConn1 -- s7/RConn1 -- OP3/LConn2
  OP3/RConn1 -- -g3/RConn1 -- s5/RConn1
  Electrical Reference3/LConn1 -- OP3/LConn1
  2/RConn1 -- s6/LConn1
  1/RConn1 -- s7/LConn1

== system onelink_simscape/summer4 ==
  Electrical Reference3 : fl_lib/Electrical/Electrical Elements/Electrical Reference
  OP3 : ee_lib/Integrated Circuits/Band-Limited Op-Amp  A=1.8E6  Rin=4e6 Ohm  Rout=70 Ohm  Vmin=-24 V  Vmax=24 V  Vdotmax=2.8E6 V/s  f=8E6 Hz  V0=0 V
  s5 : fl_lib/Electrical/Electrical Elements/Resistor  R=10E3 Ohm  i_specify=off  i_priority=None  i=0 A  i_nominal_specify=off  i_nominal_value=1  i_nominal_unit=A  v_specify=off  v_priority=None  v=0 V  v_nominal_specify=off  v_nominal_value=1  v_nominal_unit=V
  s6 : fl_lib/Electrical/Electrical Elements/Resistor  R=10E3 Ohm  i_specify=off  i_priority=None  i=0 A  i_nominal_specify=off  i_nominal_value=1  i_nominal_unit=A  v_specify=off  v_priority=None  v=0 V  v_nominal_specify=off  v_nominal_value=1  v_nominal_unit=V
  s7 : fl_lib/Electrical/Electrical Elements/Resistor  R=10E3 Ohm  i_specify=off  i_priority=None  i=0 A  i_nominal_specify=off  i_nominal_value=1  i_nominal_unit=A  v_specify=off  v_priority=None  v=0 V  v_nominal_specify=off  v_nominal_value=1  v_nominal_unit=V
  1 : PMIOPort  Side=Left
  2 : PMIOPort  Port=2  Side=Left
  -e1 : PMIOPort  Port=3  Side=Right
  connections:
  s6/RConn1 -- s5/LConn1 -- s7/RConn1 -- OP3/LConn2
  OP3/RConn1 -- -e1/RConn1 -- s5/RConn1
  Electrical Reference3/LConn1 -- OP3/LConn1
  2/RConn1 -- s6/LConn1
  1/RConn1 -- s7/LConn1

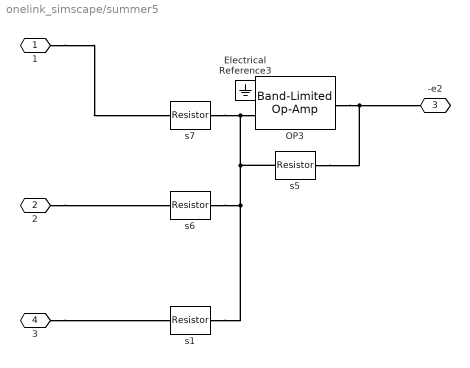
== system onelink_simscape/summer5 ==
  Electrical Reference3 : fl_lib/Electrical/Electrical Elements/Electrical Reference
  OP3 : ee_lib/Integrated Circuits/Band-Limited Op-Amp  A=1.8E6  Rin=4e6 Ohm  Rout=70 Ohm  Vmin=-24 V  Vmax=24 V  Vdotmax=2.8E6 V/s  f=8E6 Hz  V0=0 V
  s{1,5..7} (4 alike) : fl_lib/Electrical/Electrical Elements/Resistor  R=10E3 Ohm  i_specify=off  i_priority=None  i=0 A  i_nominal_specify=off  i_nominal_value=1  i_nominal_unit=A  v_specify=off  v_priority=None  v=0 V  v_nominal_specify=off  v_nominal_value=1  v_nominal_unit=V
  1 : PMIOPort  Side=Left
  2 : PMIOPort  Port=2  Side=Left
  -e2 : PMIOPort  Port=3  Side=Right
  3 : PMIOPort  Port=4  Side=Left
  connections:
  3/RConn1 -- s1/LConn1
  s1/RConn1 -- s6/RConn1 -- s5/LConn1 -- s7/RConn1 -- OP3/LConn2
  OP3/RConn1 -- -e2/RConn1 -- s5/RConn1
  Electrical Reference3/LConn1 -- OP3/LConn1
  2/RConn1 -- s6/LConn1
  1/RConn1 -- s7/LConn1

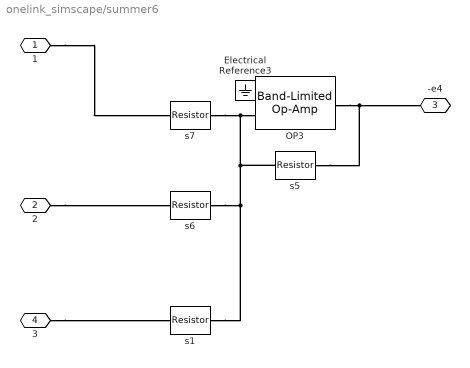
== system onelink_simscape/summer6 ==
  Electrical Reference3 : fl_lib/Electrical/Electrical Elements/Electrical Reference
  OP3 : ee_lib/Integrated Circuits/Band-Limited Op-Amp  A=1.8E6  Rin=4e6 Ohm  Rout=70 Ohm  Vmin=-24 V  Vmax=24 V  Vdotmax=2.8E6 V/s  f=8E6 Hz  V0=0 V
  s{1,5..7} (4 alike) : fl_lib/Electrical/Electrical Elements/Resistor  R=10E3 Ohm  i_specify=off  i_priority=None  i=0 A  i_nominal_specify=off  i_nominal_value=1  i_nominal_unit=A  v_specify=off  v_priority=None  v=0 V  v_nominal_specify=off  v_nominal_value=1  v_nominal_unit=V
  1 : PMIOPort  Side=Left
  2 : PMIOPort  Port=2  Side=Left
  -e4 : PMIOPort  Port=3  Side=Right
  3 : PMIOPort  Port=4  Side=Left
  connections:
  3/RConn1 -- s1/LConn1
  s1/RConn1 -- s6/RConn1 -- s5/LConn1 -- s7/RConn1 -- OP3/LConn2
  OP3/RConn1 -- -e4/RConn1 -- s5/RConn1
  Electrical Reference3/LConn1 -- OP3/LConn1
  2/RConn1 -- s6/LConn1
  1/RConn1 -- s7/LConn1

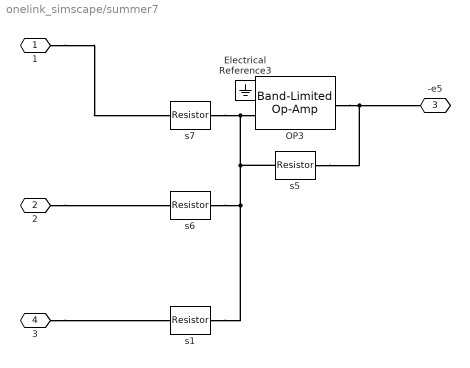
== system onelink_simscape/summer7 ==
  Electrical Reference3 : fl_lib/Electrical/Electrical Elements/Electrical Reference
  OP3 : ee_lib/Integrated Circuits/Band-Limited Op-Amp  A=1.8E6  Rin=4e6 Ohm  Rout=70 Ohm  Vmin=-24 V  Vmax=24 V  Vdotmax=2.8E6 V/s  f=8E6 Hz  V0=0 V
  s{1,5..7} (4 alike) : fl_lib/Electrical/Electrical Elements/Resistor  R=10E3 Ohm  i_specify=off  i_priority=None  i=0 A  i_nominal_specify=off  i_nominal_value=1  i_nominal_unit=A  v_specify=off  v_priority=None  v=0 V  v_nominal_specify=off  v_nominal_value=1  v_nominal_unit=V
  1 : PMIOPort  Side=Left
  2 : PMIOPort  Port=2  Side=Left
  -e5 : PMIOPort  Port=3  Side=Right
  3 : PMIOPort  Port=4  Side=Left
  connections:
  3/RConn1 -- s1/LConn1
  s1/RConn1 -- s6/RConn1 -- s5/LConn1 -- s7/RConn1 -- OP3/LConn2
  OP3/RConn1 -- -e5/RConn1 -- s5/RConn1
  Electrical Reference3/LConn1 -- OP3/LConn1
  2/RConn1 -- s6/LConn1
  1/RConn1 -- s7/LConn1

== system onelink_simscape/summer8 ==
  Electrical Reference3 : fl_lib/Electrical/Electrical Elements/Electrical Reference
  OP3 : ee_lib/Integrated Circuits/Band-Limited Op-Amp  A=1.8E6  Rin=4e6 Ohm  Rout=70 Ohm  Vmin=-24 V  Vmax=24 V  Vdotmax=2.8E6 V/s  f=8E6 Hz  V0=0 V
  s5 : fl_lib/Electrical/Electrical Elements/Resistor  R=10E3 Ohm  i_specify=off  i_priority=None  i=0 A  i_nominal_specify=off  i_nominal_value=1  i_nominal_unit=A  v_specify=off  v_priority=None  v=0 V  v_nominal_specify=off  v_nominal_value=1  v_nominal_unit=V
  s6 : fl_lib/Electrical/Electrical Elements/Resistor  R=10E3 Ohm  i_specify=off  i_priority=None  i=0 A  i_nominal_specify=off  i_nominal_value=1  i_nominal_unit=A  v_specify=off  v_priority=None  v=0 V  v_nominal_specify=off  v_nominal_value=1  v_nominal_unit=V
  s7 : fl_lib/Electrical/Electrical Elements/Resistor  R=10E3 Ohm  i_specify=off  i_priority=None  i=0 A  i_nominal_specify=off  i_nominal_value=1  i_nominal_unit=A  v_specify=off  v_priority=None  v=0 V  v_nominal_specify=off  v_nominal_value=1  v_nominal_unit=V
  1 : PMIOPort  Side=Left
  2 : PMIOPort  Port=2  Side=Left
  -g1 : PMIOPort  Port=3  Side=Right
  connections:
  s6/RConn1 -- s5/LConn1 -- s7/RConn1 -- OP3/LConn2
  OP3/RConn1 -- -g1/RConn1 -- s5/RConn1
  Electrical Reference3/LConn1 -- OP3/LConn1
  2/RConn1 -- s6/LConn1
  1/RConn1 -- s7/LConn1

== system onelink_simscape/summer9 ==
  Electrical Reference3 : fl_lib/Electrical/Electrical Elements/Electrical Reference
  OP3 : ee_lib/Integrated Circuits/Band-Limited Op-Amp  A=1.8E6  Rin=4e6 Ohm  Rout=70 Ohm  Vmin=-24 V  Vmax=24 V  Vdotmax=2.8E6 V/s  f=8E6 Hz  V0=0 V
  s5 : fl_lib/Electrical/Electrical Elements/Resistor  R=10E3 Ohm  i_specify=off  i_priority=None  i=0 A  i_nominal_specify=off  i_nominal_value=1  i_nominal_unit=A  v_specify=off  v_priority=None  v=0 V  v_nominal_specify=off  v_nominal_value=1  v_nominal_unit=V
  s6 : fl_lib/Electrical/Electrical Elements/Resistor  R=10E3 Ohm  i_specify=off  i_priority=None  i=0 A  i_nominal_specify=off  i_nominal_value=1  i_nominal_unit=A  v_specify=off  v_priority=None  v=0 V  v_nominal_specify=off  v_nominal_value=1  v_nominal_unit=V
  s7 : fl_lib/Electrical/Electrical Elements/Resistor  R=10E3 Ohm  i_specify=off  i_priority=None  i=0 A  i_nominal_specify=off  i_nominal_value=1  i_nominal_unit=A  v_specify=off  v_priority=None  v=0 V  v_nominal_specify=off  v_nominal_value=1  v_nominal_unit=V
  1 : PMIOPort  Side=Left
  2 : PMIOPort  Port=2  Side=Left
  -g4 : PMIOPort  Port=3  Side=Right
  connections:
  s6/RConn1 -- s5/LConn1 -- s7/RConn1 -- OP3/LConn2
  OP3/RConn1 -- -g4/RConn1 -- s5/RConn1
  Electrical Reference3/LConn1 -- OP3/LConn1
  2/RConn1 -- s6/LConn1
  1/RConn1 -- s7/LConn1

== system onelink_simscape/cosine converter/Sensor1 ==
  ERef : fl_lib/Electrical/Electrical Elements/Electrical Reference
  PS-Simulink Converter : nesl_utility/PS-Simulink Converter  PhysicalDomain=network_engine_domain  SubClassName=ps_output  LeftPortType=input  RightPortType=output  PseudoPeriodic=off  Frequencies=[]  VectorFormat=1-D array  Unit=1  AffineConversion=off
  Voltage Sensor : fl_lib/Electrical/Electrical Sensors/Voltage Sensor
  Conn1 : PMIOPort  Side=Left
  Out1 : Outport  VectorParamsAs1DForOutWhenUnconnected=off
  wires:
  PS-Simulink Converter/1 -> Out1/1
  connections:
  ERef/LConn1 -- Voltage Sensor/RConn2
  Voltage Sensor/RConn1 -- PS-Simulink Converter/LConn1
  Voltage Sensor/LConn1 -- Conn1/RConn1

== system onelink_simscape/sine converter1/Sensor1 ==
  ERef : fl_lib/Electrical/Electrical Elements/Electrical Reference
  PS-Simulink Converter : nesl_utility/PS-Simulink Converter  PhysicalDomain=network_engine_domain  SubClassName=ps_output  LeftPortType=input  RightPortType=output  PseudoPeriodic=off  Frequencies=[]  VectorFormat=1-D array  Unit=1  AffineConversion=off
  Voltage Sensor : fl_lib/Electrical/Electrical Sensors/Voltage Sensor
  Conn1 : PMIOPort  Side=Left
  Out1 : Outport  VectorParamsAs1DForOutWhenUnconnected=off
  wires:
  PS-Simulink Converter/1 -> Out1/1
  connections:
  Voltage Sensor/LConn1 -- Conn1/RConn1
  Voltage Sensor/RConn1 -- PS-Simulink Converter/LConn1
  ERef/LConn1 -- Voltage Sensor/RConn2
